simulink model "Just_The_Electrical_model"  (R2016a)
settings: Solver=VariableStepAuto  StartTime=0.0  StopTime=10.0  RelTol=1e-3
values from neighbouring files (symbols this model uses):
  BT = {}    [Electrical_model_settings.m]
  btc = {}    [Electrical_model_settings.m]
  col = {}    [Electrical_model_settings.m]
  elc = {}    [Electrical_model_settings.m]
  ess = {}    [Electrical_model_settings.m]
  fcc = {}    [Electrical_model_settings.m]
  flex = {}    [Electrical_model_settings.m]
  systemBase = {}    [Electrical_model_settings.m]
  wf = {}    [Electrical_model_settings.m]
  wt1 = {}    [Electrical_model_settings.m]
  wt2 = wt1    [Electrical_model_settings.m]
  wt3 = wt1    [Electrical_model_settings.m]
undefined symbols (not defined in the file or in its folder): avr, D1, Delta, DiscIntNeverNeededParam, f2ctrl, governor, interface, Lf1, sm, Ts, Ts_phy, Ts_sim, u0
libraries: powerlib x69, pwrsysBasic x68, simulink_extras x37, pwrsysVICtrl x22, powerlib_meascontrol x19, simulink x8, pwrsysVSrc x5, pwrsysTransf x5, pwrsys-matlab x1
(part 4 of 4)

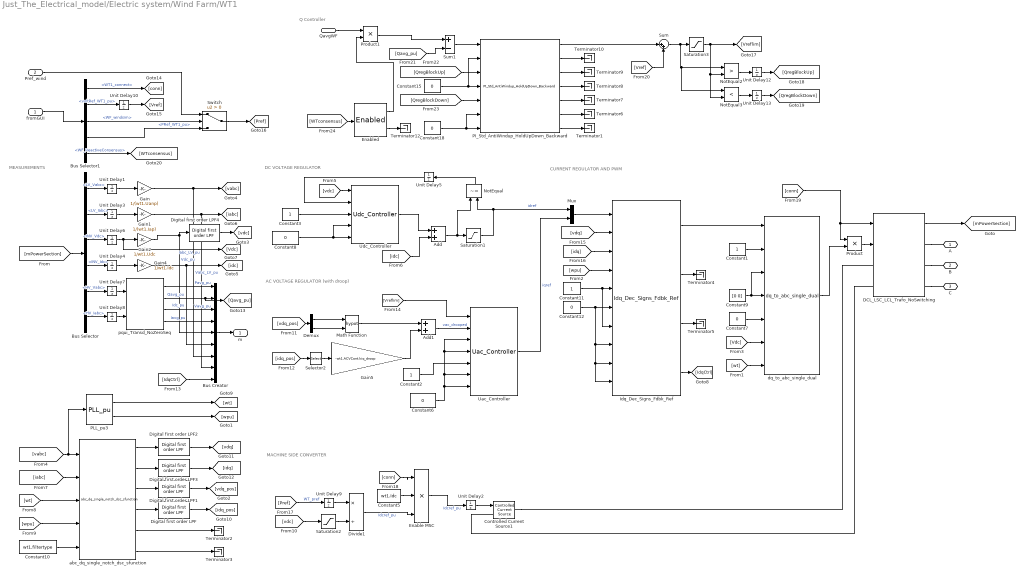
== system Just_The_Electrical_model/Electric system/Wind Farm/WT1 ==
  note: MEASUREMENTS
  note: MACHINE SIDE CONVERTER
  note: AC VOLTAGE REGULATOR (with droop)
  note: DC VOLTAGE REGULATOR
  note: CURRENT REGULATOR AND PWM
  note: Q Controller
  fromGUI : Inport
  Pref_wind : Inport  Port=2
  QavgWF : Inport  Port=3
  Add : Sum
  Add1 : Sum
  Bus Creator : BusCreator  Inputs=9
  Bus Selector : BusSelector  OutputSignals=LV_Vabc,LV_Iabc,INV_Vdc,INV_Idc,HV_Vabc,HV_Iabc
  Bus Selector1 : BusSelector  OutputSignals=WT1_connect,voltRef_WT1_pu,WF_windsim,PRef_WT1_pu,WF_ReactiveConsensus
  Constant1 : Constant  SampleTime=wt1.Ts_control
  Constant10 : Constant  Value=wt1.filtertype  SampleTime=wt1.Ts_control
  Constant11 : Constant  SampleTime=wt2.Ts_control
  Constant12 : Constant  Value=0  SampleTime=wt2.Ts_control
  Constant15 : Constant  Value=0
  Constant18 : Constant  Value=0
  Constant2 : Constant  SampleTime=wt2.Ts_control
  Constant3 : Constant  SampleTime=wt2.Ts_control
  Constant5 : Constant  Value=wt1.Idc  SampleTime=wt1.Ts_control
  Constant6 : Constant  Value=0  SampleTime=wt1.Ts_control
  Constant7 : Constant  Value=0  SampleTime=wt1.Ts_control
  Constant8 : Constant  Value=0  SampleTime=wt1.Ts_control
  Constant9 : Constant  Value=[0 0]  SampleTime=wt1.Ts_control
  Controlled Current Source1 : powerlib/Electrical Sources/Controlled Current Source  Initialize=on  Source_Type=DC  Amplitude=0  Phase=0  Frequency=50  Measurements=None
  DCL_LSC_LCL_Trafo_NoSwitching : pwrsysVSrc/DCL_LSC_LCL_Trafo_NoSwitching  Sn=wt1.Sn  fn=systemBase.fn  Uhv_ab=col.Un  Uab=wt1.Un  lf2=wt1.LCL.l2  rf2=wt1.LCL.r2  Lf1=wt1.LCL.L1  Rf1=wt1.LCL.R1  Cf=wt1.LCL.Cf  Rc=wt1.LCL.Rf  Cdc=wt1.Cdc  Udc0=wt1.Udc  Tsm=wt1.Ts_control  Tstart=wt1.DCVCont.Start
  Demux : Demux  Outputs=2
  Digital first order LPF{,1..4} (5 alike) : pwrsysBasic/Digital first order LPF  Ts=wt1.Ts_control  fcutout=wt1.CurrCont.f_LPF_noise
  Divide1 : Product  Inputs=*/
  Enable MSC : Product  Inputs=3
  Enabled : pwrsysBasic/Enabled
  Gain : Gain  Gain=1/(wt1.Uanp)
  Gain1 : Gain  Gain=1/(wt1.Iap)
  Gain2 : Gain  Gain=1/wt1.Udc
  Gain4 : Gain  Gain=1/wt1.Idc
  Gain5 : Gain  Gain=-wt1.ACVCont.kiq_droop
  Idq_Dec_Signs_Fdbk_Ref : pwrsysVICtrl/Idq_Dec_Signs_Fdbk_Ref  Ts=wt1.Ts_control  fn=systemBase.fn  Kp=wt1.CurrContSingle.kp  Ti=wt1.CurrContSingle.Ti  L=wt1.CurrCont.x  PI_max=wt1.CurrCont.PImax  PI_min=wt1.CurrCont.PImin  TrafoPhaseComp=0
  Math Function : Math  Operator=hypot  SaturateOnIntegerOverflow=on
  Mux : Mux  Inputs=2
  NotEqual : RelationalOperator  Operator=~=  OutDataTypeStr=boolean
  NotEqual2 : RelationalOperator  Operator=>  OutDataTypeStr=boolean
  NotEqual3 : RelationalOperator  Operator=<  OutDataTypeStr=boolean
  PI_Std_AntiWindup_HoldUpDown_Backward : pwrsysBasic/PI_Std_AntiWindup_HoldUpDown_Backward  Ts=wt1.Ts_control  Kg=wt1.Qctrl.Kg  Kp=wt1.Qctrl.Kp  Ti=wt1.Qctrl.Ti  outMax=wt1.Qctrl.deltaUmaxPos  outMin=wt1.Qctrl.deltaUmaxNeg
  PLL_pu3 : pwrsysBasic/PLL_pu  fn=systemBase.fn  Ts=wt1.Ts_control  Kp_pll=90  Ki_pll=1200  Kd_pll=0  PLL_ini=60
  Product : Product
  Product1 : Product
  Saturation1 : Saturate  UpperLimit=wt1.DCVCont.PImax  LowerLimit=wt1.DCVCont.PImin
  Saturation2 : Saturate  UpperLimit=1.2  LowerLimit=0.8
  Saturation3 : Saturate  UpperLimit=wt1.Qctrl.Umax  LowerLimit=wt1.Qctrl.Umin
  Selector2 : Selector  IndexMode=Zero-based  InputPortWidth=2  IndexOptions=Index vector (dialog)  Indices=1  OutputSizes=1
  Sum : Sum  Inputs=|++
  Sum1 : Sum  Inputs=+-
  Switch : Switch  Criteria=u2 > Threshold
  Terminator{1..10,12} (11 alike) : Terminator
  Uac_Controller : pwrsysVICtrl/Uac_Controller  Ts=wt1.Ts_control  Kg=wt1.ACVCont.kg  Kp=wt1.ACVCont.kp  Ti=wt1.ACVCont.Ti  PI_max=wt1.ACVCont.PImax  PI_min=wt1.ACVCont.PImin
  Udc_Controller : pwrsysVICtrl/Udc_Controller  Ts=wt1.Ts_control  Kp=wt1.DCVContSingle.kp  Ti=wt1.DCVContSingle.Ti  PI_max=wt1.DCVCont.PImax  PI_min=wt1.DCVCont.PImin
  Unit Delay{1,3,7..8} (4 alike) : UnitDelay  InitialCondition=[0 0 0]  SampleTime=wt1.Ts_control
  Unit Delay10 : UnitDelay  InitialCondition=1  SampleTime=wt1.Ts_control
  Unit Delay{2,4..5,9,12..13} (6 alike) : UnitDelay  SampleTime=wt1.Ts_control
  Unit Delay6 : UnitDelay  InitialCondition=1  SampleTime=wt1.Ts_control
  abc_dq_single_notch_dsc_sfunction : pwrsysTransf/abc_dq_single_notch_dsc_sfunction  Ts=wt1.Ts_control  fn=2*systemBase.fn  zeta=wt1.CurrCont.zeta
  dq_to_abc_single_dual : pwrsysVICtrl/dq_to_abc_single_dual  Ts=wt1.Ts_control  Uabp=wt1.Uabp
  pqui_Transd_NoZeroSeq : pwrsysBasic/pqui_Transd_NoZeroSeq  Sn=wt1.Sn  Uanp=col.Uanp  Iap=wt1.Iap*(wt1.Un/col.Un)
  A : PMIOPort  Port=1  Side=Right
  B : PMIOPort  Port=2  Side=Right
  C : PMIOPort  Port=3  Side=Right
  m : Outport
  wires:
  Divide1/1 -> Enable MSC/3  "Idcref_pu"
  Bus Selector/1 -> Unit Delay1/1  "<LV_Vabc>"
  [idq_pos] -> Selector2/1
  Unit Delay2/1 -> Controlled Current Source1/1
  Gain1/1 -> Bus Creator/8, [iabc]  "Iabc_LV_pu"
  Bus Selector/2 -> Unit Delay3/1  "<LV_Iabc>"
  Gain5/1 -> Add1/2
  Math Function/1 -> Add1/1
  Constant6/1 -> Uac_Controller/7, Uac_Controller/6, Uac_Controller/3, Uac_Controller/4
  Constant5/1 -> Enable MSC/2
  Add1/1 -> Uac_Controller/2  "vac_drooped"
  [mPowerSection] -> Bus Selector/1
  Enable MSC/1 -> Unit Delay2/1  "Idcref_pu"
  Gain/1 -> Bus Creator/7, [vabc]  "Vabc_LV_pu"
  Constant2/1 -> Uac_Controller/5
  Constant8/1 -> Udc_Controller/4, Udc_Controller/5
  NotEqual/1 -> Unit Delay5/1
  [vdc] -> Udc_Controller/1
  Unit Delay5/1 -> Udc_Controller/2
  Saturation1/1 -> NotEqual/2, Mux/1  "idref"
  [idc] -> Add/2
  Udc_Controller/1 -> Add/1
  Add/1 -> NotEqual/1, Saturation1/1
  Constant3/1 -> Udc_Controller/3
  [idq] -> Idq_Dec_Signs_Fdbk_Ref/3
  [Vdc] -> dq_to_abc_single_dual/6
  [wpu] -> Idq_Dec_Signs_Fdbk_Ref/4
  dq_to_abc_single_dual/1 -> Product/2
  [conn] -> Product/1, DCL_LSC_LCL_Trafo_NoSwitching/1
  Saturation2/1 -> Divide1/2
  [Pref] -> Unit Delay9/1  "WT_pref"
  [vdc] -> Saturation2/1
  [wt] -> dq_to_abc_single_dual/7
  Constant10/1 -> abc_dq_single_notch_dsc_sfunction/5
  Bus Selector/5 -> Unit Delay7/1  "<HV_Vabc>"
  Bus Selector/6 -> Unit Delay8/1  "<HV_Iabc>"
  pqui_Transd_NoZeroSeq/1 -> Bus Creator/1  "Pavg_pu"
  pqui_Transd_NoZeroSeq/2 -> [Qavg_pu], Bus Creator/2  "Qavg_pu"
  pqui_Transd_NoZeroSeq/3 -> Bus Creator/3  "Vavg_pu"
  pqui_Transd_NoZeroSeq/4 -> Bus Creator/4  "Iavg_pu"
  Bus Creator/1 -> m/1
  Bus Selector/3 -> Unit Delay6/1  "<INV_Vdc>"
  Gain2/1 -> Digital first order LPF4/1, Bus Creator/5  "Vdc_pu"
  Gain4/1 -> [idc], Bus Creator/6  "Idc_pu"
  Bus Selector/4 -> Unit Delay4/1  "<INV_Idc>"
  PLL_pu3/2 -> [wpu]
  PLL_pu3/1 -> [wt]
  Uac_Controller/1 -> Mux/2  "iqref"
  DCL_LSC_LCL_Trafo_NoSwitching/1 -> [mPowerSection]
  Unit Delay1/1 -> Gain/1
  Unit Delay3/1 -> Gain1/1
  Unit Delay4/1 -> Gain4/1
  Unit Delay8/1 -> pqui_Transd_NoZeroSeq/2
  Unit Delay6/1 -> [Vdc], Gain2/1
  Unit Delay7/1 -> pqui_Transd_NoZeroSeq/1
  Unit Delay9/1 -> Divide1/1
  [Vreflim] -> Uac_Controller/1
  abc_dq_single_notch_dsc_sfunction/6 -> Terminator3/1
  abc_dq_single_notch_dsc_sfunction/5 -> Terminator2/1
  Selector2/1 -> Gain5/1
  Idq_Dec_Signs_Fdbk_Ref/2 -> Terminator4/1
  [vdq] -> Idq_Dec_Signs_Fdbk_Ref/2
  Constant1/1 -> dq_to_abc_single_dual/2
  Constant7/1 -> dq_to_abc_single_dual/5
  Constant9/1 -> dq_to_abc_single_dual/4, dq_to_abc_single_dual/3
  Constant11/1 -> Idq_Dec_Signs_Fdbk_Ref/7, Idq_Dec_Signs_Fdbk_Ref/5
  Constant12/1 -> Idq_Dec_Signs_Fdbk_Ref/8, Idq_Dec_Signs_Fdbk_Ref/9, Idq_Dec_Signs_Fdbk_Ref/10, Idq_Dec_Signs_Fdbk_Ref/6
  Idq_Dec_Signs_Fdbk_Ref/3 -> Terminator5/1
  Idq_Dec_Signs_Fdbk_Ref/4 -> [IdqCtrl]
  [IdqCtrl] -> Bus Creator/9
  Idq_Dec_Signs_Fdbk_Ref/1 -> dq_to_abc_single_dual/1
  [wt] -> abc_dq_single_notch_dsc_sfunction/3
  [wpu] -> abc_dq_single_notch_dsc_sfunction/4
  abc_dq_single_notch_dsc_sfunction/1 -> Digital first order LPF2/1
  [vabc] -> abc_dq_single_notch_dsc_sfunction/1, PLL_pu3/1
  [iabc] -> abc_dq_single_notch_dsc_sfunction/2
  abc_dq_single_notch_dsc_sfunction/3 -> Digital first order LPF1/1
  abc_dq_single_notch_dsc_sfunction/4 -> Digital first order LPF/1
  abc_dq_single_notch_dsc_sfunction/2 -> Digital first order LPF3/1
  Digital first order LPF/1 -> [idq_pos]
  Digital first order LPF1/1 -> [vdq_pos]
  [vdq_pos] -> Demux/1
  Demux/1 -> Math Function/1
  Demux/2 -> Math Function/2
  Digital first order LPF2/1 -> [vdq]
  Digital first order LPF3/1 -> [idq]
  Digital first order LPF4/1 -> [vdc]
  fromGUI/1 -> Bus Selector1/1
  Bus Selector1/4 -> Switch/3  "<PRef_WT1_pu>"
  Bus Selector1/1 -> [conn]  "<WT1_connect>"
  Bus Selector1/2 -> Unit Delay10/1  "<voltRef_WT1_pu>"
  [conn] -> Enable MSC/1
  Pref_wind/1 -> Switch/1
  Bus Selector1/3 -> Switch/2  "<WF_windsim>"
  Switch/1 -> [Pref]
  Mux/1 -> Idq_Dec_Signs_Fdbk_Ref/1
  Product/1 -> DCL_LSC_LCL_Trafo_NoSwitching/2
  Unit Delay10/1 -> [Vref]
  [Vref] -> Sum/2
  Sum/1 -> NotEqual3/1, NotEqual2/1, Saturation3/1
  Saturation3/1 -> NotEqual3/2, NotEqual2/2, [Vreflim]
  [Qavg_pu] -> Sum1/2
  [WTconsensus] -> Enabled/1
  [QregBlockUp] -> PI_Std_AntiWindup_HoldUpDown_Backward/3
  Constant15/1 -> PI_Std_AntiWindup_HoldUpDown_Backward/2, PI_Std_AntiWindup_HoldUpDown_Backward/4
  [QregBlockDown] -> PI_Std_AntiWindup_HoldUpDown_Backward/5
  Constant18/1 -> PI_Std_AntiWindup_HoldUpDown_Backward/6, PI_Std_AntiWindup_HoldUpDown_Backward/7
  PI_Std_AntiWindup_HoldUpDown_Backward/7 -> Terminator1/1
  PI_Std_AntiWindup_HoldUpDown_Backward/6 -> Terminator6/1
  PI_Std_AntiWindup_HoldUpDown_Backward/5 -> Terminator7/1
  PI_Std_AntiWindup_HoldUpDown_Backward/4 -> Terminator8/1
  PI_Std_AntiWindup_HoldUpDown_Backward/3 -> Terminator9/1
  PI_Std_AntiWindup_HoldUpDown_Backward/2 -> Terminator10/1
  NotEqual2/1 -> Unit Delay12/1
  Unit Delay12/1 -> [QregBlockUp]
  NotEqual3/1 -> Unit Delay13/1
  Unit Delay13/1 -> [QregBlockDown]
  PI_Std_AntiWindup_HoldUpDown_Backward/1 -> Sum/1
  Bus Selector1/5 -> [WTconsensus]  "<WF_ReactiveConsensus>"
  Sum1/1 -> PI_Std_AntiWindup_HoldUpDown_Backward/1
  Enabled/2 -> Terminator12/1
  QavgWF/1 -> Product1/1
  Product1/1 -> Sum1/1
  Enabled/1 -> Product1/2
  connections:
  Controlled Current Source1/RConn1 -- DCL_LSC_LCL_Trafo_NoSwitching/LConn1
  DCL_LSC_LCL_Trafo_NoSwitching/RConn3 -- C/RConn1
  DCL_LSC_LCL_Trafo_NoSwitching/RConn1 -- A/RConn1
  DCL_LSC_LCL_Trafo_NoSwitching/RConn2 -- B/RConn1
  Controlled Current Source1/LConn1 -- DCL_LSC_LCL_Trafo_NoSwitching/LConn2

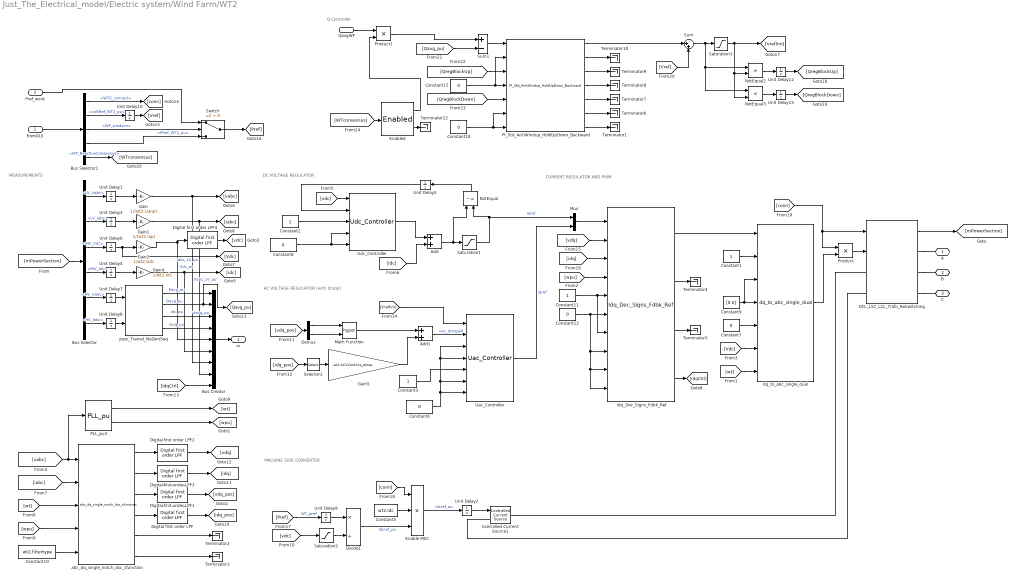
== system Just_The_Electrical_model/Electric system/Wind Farm/WT2 ==
  note: MEASUREMENTS
  note: MACHINE SIDE CONVERTER
  note: AC VOLTAGE REGULATOR (with droop)
  note: DC VOLTAGE REGULATOR
  note: CURRENT REGULATOR AND PWM
  note: Q Controller
  fromGUI : Inport
  Pref_wind : Inport  Port=2
  QavgWF : Inport  Port=3
  Add : Sum
  Add1 : Sum
  Bus Creator : BusCreator  Inputs=9
  Bus Selector : BusSelector  OutputSignals=LV_Vabc,LV_Iabc,INV_Vdc,INV_Idc,HV_Vabc,HV_Iabc
  Bus Selector1 : BusSelector  OutputSignals=WT2_connect,voltRef_WT2_pu,WF_windsim,PRef_WT2_pu,WF_ReactiveConsensus
  Constant{1..3,11} (4 alike) : Constant  SampleTime=wt2.Ts_control
  Constant10 : Constant  Value=wt2.filtertype  SampleTime=wt2.Ts_control
  Constant{6..8,12} (4 alike) : Constant  Value=0  SampleTime=wt2.Ts_control
  Constant15 : Constant  Value=0
  Constant18 : Constant  Value=0
  Constant5 : Constant  Value=wt2.Idc  SampleTime=wt2.Ts_control
  Constant9 : Constant  Value=[0 0]  SampleTime=wt2.Ts_control
  Controlled Current Source1 : powerlib/Electrical Sources/Controlled Current Source  Initialize=on  Source_Type=DC  Amplitude=0  Phase=0  Frequency=50  Measurements=None
  DCL_LSC_LCL_Trafo_NoSwitching : pwrsysVSrc/DCL_LSC_LCL_Trafo_NoSwitching  Sn=wt2.Sn  fn=systemBase.fn  Uhv_ab=col.Un  Uab=wt2.Un  lf2=wt2.LCL.l2  rf2=wt2.LCL.r2  Lf1=wt2.LCL.L1  Rf1=wt2.LCL.R1  Cf=wt2.LCL.Cf  Rc=wt2.LCL.Rf  Cdc=wt2.Cdc  Udc0=wt2.Udc  Tsm=wt2.Ts_control  Tstart=wt2.DCVCont.Start
  Demux : Demux  Outputs=2
  Digital first order LPF{,1..4} (5 alike) : pwrsysBasic/Digital first order LPF  Ts=wt2.Ts_control  fcutout=wt2.CurrCont.f_LPF_noise
  Divide1 : Product  Inputs=*/
  Enable MSC : Product  Inputs=3
  Enabled : pwrsysBasic/Enabled
  Gain : Gain  Gain=1/(wt2.Uanp)
  Gain1 : Gain  Gain=1/(wt2.Iap)
  Gain2 : Gain  Gain=1/wt2.Udc
  Gain4 : Gain  Gain=1/wt2.Idc
  Gain5 : Gain  Gain=-wt2.ACVCont.kiq_droop
  Idq_Dec_Signs_Fdbk_Ref : pwrsysVICtrl/Idq_Dec_Signs_Fdbk_Ref  Ts=wt2.Ts_control  fn=systemBase.fn  Kp=wt2.CurrContSingle.kp  Ti=wt2.CurrContSingle.Ti  L=wt2.CurrCont.x  PI_max=wt2.CurrCont.PImax  PI_min=wt2.CurrCont.PImin  TrafoPhaseComp=0
  Math Function : Math  Operator=hypot  SaturateOnIntegerOverflow=on
  Mux : Mux  Inputs=2
  NotEqual : RelationalOperator  Operator=~=  OutDataTypeStr=boolean
  NotEqual2 : RelationalOperator  Operator=>  OutDataTypeStr=boolean
  NotEqual3 : RelationalOperator  Operator=<  OutDataTypeStr=boolean
  PI_Std_AntiWindup_HoldUpDown_Backward : pwrsysBasic/PI_Std_AntiWindup_HoldUpDown_Backward  Ts=wt2.Ts_control  Kg=wt2.Qctrl.Kg  Kp=wt2.Qctrl.Kp  Ti=wt2.Qctrl.Ti  outMax=wt2.Qctrl.deltaUmaxPos  outMin=wt2.Qctrl.deltaUmaxNeg
  PLL_pu3 : pwrsysBasic/PLL_pu  fn=systemBase.fn  Ts=wt2.Ts_control  Kp_pll=90  Ki_pll=1200  Kd_pll=0  PLL_ini=60
  Product : Product
  Product1 : Product
  Saturation1 : Saturate  UpperLimit=wt2.DCVCont.PImax  LowerLimit=wt2.DCVCont.PImin
  Saturation2 : Saturate  UpperLimit=1.2  LowerLimit=0.8
  Saturation3 : Saturate  UpperLimit=wt2.Qctrl.Umax  LowerLimit=wt2.Qctrl.Umin
  Selector2 : Selector  IndexMode=Zero-based  InputPortWidth=2  IndexOptions=Index vector (dialog)  Indices=1  OutputSizes=1
  Sum : Sum  Inputs=|++
  Sum1 : Sum  Inputs=+-
  Switch : Switch  Criteria=u2 > Threshold
  Terminator{1..10,12} (11 alike) : Terminator
  Uac_Controller : pwrsysVICtrl/Uac_Controller  Ts=wt2.Ts_control  Kg=wt2.ACVCont.kg  Kp=wt2.ACVCont.kp  Ti=wt2.ACVCont.Ti  PI_max=wt2.ACVCont.PImax  PI_min=wt2.ACVCont.PImin
  Udc_Controller : pwrsysVICtrl/Udc_Controller  Ts=wt2.Ts_control  Kp=wt2.DCVContDual.kp  Ti=wt2.DCVContDual.Ti  PI_max=wt2.DCVCont.PImax  PI_min=wt2.DCVCont.PImin
  Unit Delay{1,3,7..8} (4 alike) : UnitDelay  InitialCondition=[0 0 0]  SampleTime=wt2.Ts_control
  Unit Delay10 : UnitDelay  InitialCondition=1  SampleTime=wt2.Ts_control
  Unit Delay{2,4..5,9,12..13} (6 alike) : UnitDelay  SampleTime=wt2.Ts_control
  Unit Delay6 : UnitDelay  InitialCondition=1  SampleTime=wt2.Ts_control
  abc_dq_single_notch_dsc_sfunction : pwrsysTransf/abc_dq_single_notch_dsc_sfunction  Ts=wt2.Ts_control  fn=2*systemBase.fn  zeta=wt2.CurrCont.zeta
  dq_to_abc_single_dual : pwrsysVICtrl/dq_to_abc_single_dual  Ts=wt2.Ts_control  Uabp=wt2.Uabp
  pqui_Transd_NoZeroSeq : pwrsysBasic/pqui_Transd_NoZeroSeq  Sn=wt2.Sn  Uanp=col.Uanp  Iap=wt2.Iap*(wt2.Un/col.Un)
  A : PMIOPort  Port=1  Side=Right
  B : PMIOPort  Port=2  Side=Right
  C : PMIOPort  Port=3  Side=Right
  m : Outport
  wires:
  Divide1/1 -> Enable MSC/3  "Idcref_pu"
  Bus Selector/1 -> Unit Delay1/1  "<LV_Vabc>"
  [idq_pos] -> Selector2/1
  Unit Delay2/1 -> Controlled Current Source1/1
  Gain1/1 -> Bus Creator/8, [iabc]  "Iabc_LV_pu"
  Bus Selector/2 -> Unit Delay3/1  "<LV_Iabc>"
  Gain5/1 -> Add1/2
  Math Function/1 -> Add1/1
  Constant6/1 -> Uac_Controller/7, Uac_Controller/6, Uac_Controller/3, Uac_Controller/4
  Constant5/1 -> Enable MSC/2
  Add1/1 -> Uac_Controller/2  "vac_drooped"
  [mPowerSection] -> Bus Selector/1
  Enable MSC/1 -> Unit Delay2/1  "Idcref_pu"
  Gain/1 -> Bus Creator/7, [vabc]  "Vabc_LV_pu"
  Constant3/1 -> Uac_Controller/5
  Constant8/1 -> Udc_Controller/4, Udc_Controller/5
  NotEqual/1 -> Unit Delay5/1
  [vdc] -> Udc_Controller/1
  Unit Delay5/1 -> Udc_Controller/2
  Saturation1/1 -> NotEqual/2, Mux/1  "idref"
  [idc] -> Add/2
  Udc_Controller/1 -> Add/1
  Add/1 -> NotEqual/1, Saturation1/1
  Constant2/1 -> Udc_Controller/3
  [idq] -> Idq_Dec_Signs_Fdbk_Ref/3
  [Vdc] -> dq_to_abc_single_dual/6
  [wpu] -> Idq_Dec_Signs_Fdbk_Ref/4
  dq_to_abc_single_dual/1 -> Product/2
  Mux/1 -> Idq_Dec_Signs_Fdbk_Ref/1
  [conn] -> Product/1, DCL_LSC_LCL_Trafo_NoSwitching/1
  Saturation2/1 -> Divide1/2
  [Pref] -> Unit Delay9/1  "WT_pref"
  [vdc] -> Saturation2/1
  [wt] -> dq_to_abc_single_dual/7
  Constant10/1 -> abc_dq_single_notch_dsc_sfunction/5
  Bus Selector/5 -> Unit Delay7/1  "<HV_Vabc>"
  Bus Selector/6 -> Unit Delay8/1  "<HV_Iabc>"
  pqui_Transd_NoZeroSeq/1 -> Bus Creator/1  "Pavg_pu"
  pqui_Transd_NoZeroSeq/2 -> [Qavg_pu], Bus Creator/2  "Qavg_pu"
  pqui_Transd_NoZeroSeq/3 -> Bus Creator/3  "Vavg_pu"
  pqui_Transd_NoZeroSeq/4 -> Bus Creator/4  "Iavg_pu"
  Bus Creator/1 -> m/1
  Bus Selector/3 -> Unit Delay6/1  "<INV_Vdc>"
  Gain2/1 -> Bus Creator/5, Digital first order LPF4/1  "Vdc_pu"
  Gain4/1 -> [idc], Bus Creator/6  "Idc_pu"
  Bus Selector/4 -> Unit Delay4/1  "<INV_Idc>"
  PLL_pu3/2 -> [wpu]
  PLL_pu3/1 -> [wt]
  Uac_Controller/1 -> Mux/2  "iqref"
  DCL_LSC_LCL_Trafo_NoSwitching/1 -> [mPowerSection]
  Unit Delay1/1 -> Gain/1
  Unit Delay3/1 -> Gain1/1
  Unit Delay4/1 -> Gain4/1
  Unit Delay8/1 -> pqui_Transd_NoZeroSeq/2
  Unit Delay6/1 -> [Vdc], Gain2/1
  Unit Delay7/1 -> pqui_Transd_NoZeroSeq/1
  Unit Delay9/1 -> Divide1/1
  [Vreflim] -> Uac_Controller/1
  abc_dq_single_notch_dsc_sfunction/6 -> Terminator3/1
  abc_dq_single_notch_dsc_sfunction/5 -> Terminator2/1
  Selector2/1 -> Gain5/1
  Idq_Dec_Signs_Fdbk_Ref/2 -> Terminator4/1
  [vdq] -> Idq_Dec_Signs_Fdbk_Ref/2
  Constant1/1 -> dq_to_abc_single_dual/2
  Constant7/1 -> dq_to_abc_single_dual/5
  Constant9/1 -> dq_to_abc_single_dual/4, dq_to_abc_single_dual/3
  Constant11/1 -> Idq_Dec_Signs_Fdbk_Ref/7, Idq_Dec_Signs_Fdbk_Ref/5
  Constant12/1 -> Idq_Dec_Signs_Fdbk_Ref/8, Idq_Dec_Signs_Fdbk_Ref/9, Idq_Dec_Signs_Fdbk_Ref/10, Idq_Dec_Signs_Fdbk_Ref/6
  Idq_Dec_Signs_Fdbk_Ref/3 -> Terminator5/1
  Idq_Dec_Signs_Fdbk_Ref/4 -> [IdqCtrl]
  [IdqCtrl] -> Bus Creator/9
  Idq_Dec_Signs_Fdbk_Ref/1 -> dq_to_abc_single_dual/1
  [wt] -> abc_dq_single_notch_dsc_sfunction/3
  [wpu] -> abc_dq_single_notch_dsc_sfunction/4
  abc_dq_single_notch_dsc_sfunction/1 -> Digital first order LPF2/1
  [vabc] -> abc_dq_single_notch_dsc_sfunction/1, PLL_pu3/1
  [iabc] -> abc_dq_single_notch_dsc_sfunction/2
  abc_dq_single_notch_dsc_sfunction/3 -> Digital first order LPF1/1
  abc_dq_single_notch_dsc_sfunction/4 -> Digital first order LPF/1
  abc_dq_single_notch_dsc_sfunction/2 -> Digital first order LPF3/1
  Digital first order LPF/1 -> [idq_pos]
  Digital first order LPF1/1 -> [vdq_pos]
  [vdq_pos] -> Demux/1
  Demux/1 -> Math Function/1
  Demux/2 -> Math Function/2
  Digital first order LPF2/1 -> [vdq]
  Digital first order LPF3/1 -> [idq]
  Digital first order LPF4/1 -> [vdc]
  fromGUI/1 -> Bus Selector1/1
  Bus Selector1/4 -> Switch/3  "<PRef_WT2_pu>"
  Bus Selector1/1 -> [conn]  "<WT2_connect>"
  Bus Selector1/2 -> Unit Delay10/1  "<voltRef_WT2_pu>"
  [conn] -> Enable MSC/1
  Pref_wind/1 -> Switch/1
  Bus Selector1/3 -> Switch/2  "<WF_windsim>"
  Switch/1 -> [Pref]
  Product/1 -> DCL_LSC_LCL_Trafo_NoSwitching/2
  Unit Delay10/1 -> [Vref]
  [Vref] -> Sum/2
  Sum/1 -> NotEqual3/1, NotEqual2/1, Saturation3/1
  Saturation3/1 -> NotEqual3/2, NotEqual2/2, [Vreflim]
  [Qavg_pu] -> Sum1/2
  [WTconsensus] -> Enabled/1
  [QregBlockUp] -> PI_Std_AntiWindup_HoldUpDown_Backward/3
  Constant15/1 -> PI_Std_AntiWindup_HoldUpDown_Backward/2, PI_Std_AntiWindup_HoldUpDown_Backward/4
  [QregBlockDown] -> PI_Std_AntiWindup_HoldUpDown_Backward/5
  Constant18/1 -> PI_Std_AntiWindup_HoldUpDown_Backward/6, PI_Std_AntiWindup_HoldUpDown_Backward/7
  PI_Std_AntiWindup_HoldUpDown_Backward/7 -> Terminator1/1
  PI_Std_AntiWindup_HoldUpDown_Backward/6 -> Terminator6/1
  PI_Std_AntiWindup_HoldUpDown_Backward/5 -> Terminator7/1
  PI_Std_AntiWindup_HoldUpDown_Backward/4 -> Terminator8/1
  PI_Std_AntiWindup_HoldUpDown_Backward/3 -> Terminator9/1
  PI_Std_AntiWindup_HoldUpDown_Backward/2 -> Terminator10/1
  NotEqual2/1 -> Unit Delay12/1
  Unit Delay12/1 -> [QregBlockUp]
  NotEqual3/1 -> Unit Delay13/1
  Unit Delay13/1 -> [QregBlockDown]
  PI_Std_AntiWindup_HoldUpDown_Backward/1 -> Sum/1
  Bus Selector1/5 -> [WTconsensus]  "<WF_ReactiveConsensus>"
  Sum1/1 -> PI_Std_AntiWindup_HoldUpDown_Backward/1
  Enabled/2 -> Terminator12/1
  QavgWF/1 -> Product1/1
  Product1/1 -> Sum1/1
  Enabled/1 -> Product1/2
  connections:
  Controlled Current Source1/RConn1 -- DCL_LSC_LCL_Trafo_NoSwitching/LConn1
  DCL_LSC_LCL_Trafo_NoSwitching/RConn3 -- C/RConn1
  DCL_LSC_LCL_Trafo_NoSwitching/RConn1 -- A/RConn1
  DCL_LSC_LCL_Trafo_NoSwitching/RConn2 -- B/RConn1
  Controlled Current Source1/LConn1 -- DCL_LSC_LCL_Trafo_NoSwitching/LConn2

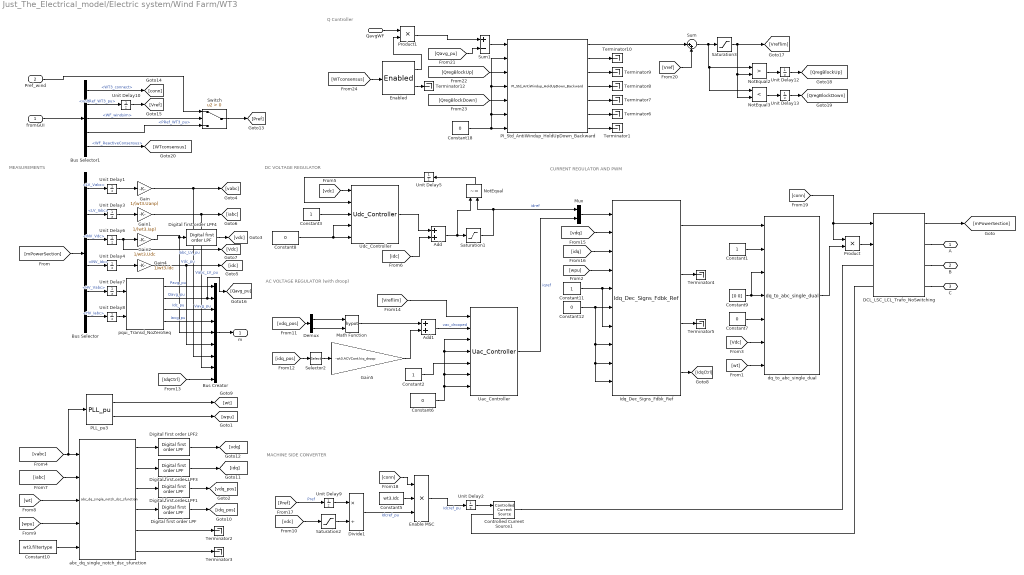
== system Just_The_Electrical_model/Electric system/Wind Farm/WT3 ==
  note: Q Controller
  note: MEASUREMENTS
  note: MACHINE SIDE CONVERTER
  note: AC VOLTAGE REGULATOR (with droop)
  note: DC VOLTAGE REGULATOR
  note: CURRENT REGULATOR AND PWM
  fromGUI : Inport
  Pref_wind : Inport  Port=2
  QavgWF : Inport  Port=3
  Add : Sum
  Add1 : Sum
  Bus Creator : BusCreator  Inputs=9
  Bus Selector : BusSelector  OutputSignals=LV_Vabc,LV_Iabc,INV_Vdc,INV_Idc,HV_Vabc,HV_Iabc
  Bus Selector1 : BusSelector  OutputSignals=WT3_connect,voltRef_WT3_pu,WF_windsim,PRef_WT3_pu,WF_ReactiveConsensus
  Constant1 : Constant  SampleTime=wt3.Ts_control
  Constant10 : Constant  Value=wt3.filtertype  SampleTime=wt3.Ts_control
  Constant11 : Constant  SampleTime=wt3.Ts_control
  Constant{6..8,12} (4 alike) : Constant  Value=0  SampleTime=wt3.Ts_control
  Constant18 : Constant  Value=0
  Constant2 : Constant  SampleTime=wt2.Ts_control
  Constant3 : Constant  SampleTime=wt2.Ts_control
  Constant5 : Constant  Value=wt3.Idc  SampleTime=wt3.Ts_control
  Constant9 : Constant  Value=[0 0]  SampleTime=wt3.Ts_control
  Controlled Current Source1 : powerlib/Electrical Sources/Controlled Current Source  Initialize=on  Source_Type=DC  Amplitude=0  Phase=0  Frequency=50  Measurements=None
  DCL_LSC_LCL_Trafo_NoSwitching : pwrsysVSrc/DCL_LSC_LCL_Trafo_NoSwitching  Sn=wt3.Sn  fn=systemBase.fn  Uhv_ab=col.Un  Uab=wt3.Un  lf2=wt3.LCL.l2  rf2=wt3.LCL.r2  Lf1=wt3.LCL.L1  Rf1=wt3.LCL.R1  Cf=wt3.LCL.Cf  Rc=wt3.LCL.Rf  Cdc=wt3.Cdc  Udc0=wt3.Udc  Tsm=wt3.Ts_control  Tstart=wt3.DCVCont.Start
  Demux : Demux  Outputs=2
  Digital first order LPF{,1..4} (5 alike) : pwrsysBasic/Digital first order LPF  Ts=wt3.Ts_control  fcutout=wt3.CurrCont.f_LPF_noise
  Divide1 : Product  Inputs=*/
  Enable MSC : Product  Inputs=***
  Enabled : pwrsysBasic/Enabled
  Gain : Gain  Gain=1/(wt3.Uanp)
  Gain1 : Gain  Gain=1/(wt3.Iap)
  Gain2 : Gain  Gain=1/wt3.Udc
  Gain4 : Gain  Gain=1/wt3.Idc
  Gain5 : Gain  Gain=-wt3.ACVCont.kiq_droop
  Idq_Dec_Signs_Fdbk_Ref : pwrsysVICtrl/Idq_Dec_Signs_Fdbk_Ref  Ts=wt3.Ts_control  fn=systemBase.fn  Kp=wt3.CurrContSingle.kp  Ti=wt3.CurrContSingle.Ti  L=wt3.CurrCont.x  PI_max=wt3.CurrCont.PImax  PI_min=wt3.CurrCont.PImin  TrafoPhaseComp=0
  Math Function : Math  Operator=hypot  SaturateOnIntegerOverflow=on
  Mux : Mux  Inputs=2
  NotEqual : RelationalOperator  Operator=~=  OutDataTypeStr=boolean
  NotEqual2 : RelationalOperator  Operator=>  OutDataTypeStr=boolean
  NotEqual3 : RelationalOperator  Operator=<  OutDataTypeStr=boolean
  PI_Std_AntiWindup_HoldUpDown_Backward : pwrsysBasic/PI_Std_AntiWindup_HoldUpDown_Backward  Ts=wt3.Ts_control  Kg=wt3.Qctrl.Kg  Kp=wt3.Qctrl.Kp  Ti=wt3.Qctrl.Ti  outMax=wt3.Qctrl.deltaUmaxPos  outMin=wt3.Qctrl.deltaUmaxNeg
  PLL_pu3 : pwrsysBasic/PLL_pu  fn=systemBase.fn  Ts=wt3.Ts_control  Kp_pll=90  Ki_pll=1200  Kd_pll=0  PLL_ini=60
  Product : Product
  Product1 : Product
  Saturation1 : Saturate  UpperLimit=wt3.DCVCont.PImax  LowerLimit=wt3.DCVCont.PImin
  Saturation2 : Saturate  UpperLimit=1.2  LowerLimit=0.8
  Saturation3 : Saturate  UpperLimit=wt3.Qctrl.Umax  LowerLimit=wt3.Qctrl.Umin
  Selector2 : Selector  IndexMode=Zero-based  InputPortWidth=2  IndexOptions=Index vector (dialog)  Indices=1  OutputSizes=1
  Sum : Sum  Inputs=|++
  Sum1 : Sum  Inputs=+-
  Switch : Switch  Criteria=u2 > Threshold
  Terminator{1..10,12} (11 alike) : Terminator
  Uac_Controller : pwrsysVICtrl/Uac_Controller  Ts=wt3.Ts_control  Kg=wt3.ACVCont.kg  Kp=wt3.ACVCont.kp  Ti=wt3.ACVCont.Ti  PI_max=wt3.ACVCont.PImax  PI_min=wt3.ACVCont.PImin
  Udc_Controller : pwrsysVICtrl/Udc_Controller  Ts=wt3.Ts_control  Kp=wt3.DCVContDual.kp  Ti=wt3.DCVContDual.Ti  PI_max=wt3.DCVCont.PImax  PI_min=wt3.DCVCont.PImin
  Unit Delay{1,3,7..8} (4 alike) : UnitDelay  InitialCondition=[0 0 0]  SampleTime=wt3.Ts_control
  Unit Delay10 : UnitDelay  InitialCondition=1  SampleTime=wt3.Ts_control
  Unit Delay{2,4..5,9,12..13} (6 alike) : UnitDelay  SampleTime=wt3.Ts_control
  Unit Delay6 : UnitDelay  InitialCondition=1  SampleTime=wt3.Ts_control
  abc_dq_single_notch_dsc_sfunction : pwrsysTransf/abc_dq_single_notch_dsc_sfunction  Ts=wt3.Ts_control  fn=2*systemBase.fn  zeta=wt3.CurrCont.zeta
  dq_to_abc_single_dual : pwrsysVICtrl/dq_to_abc_single_dual  Ts=wt3.Ts_control  Uabp=wt3.Uabp
  pqui_Transd_NoZeroSeq : pwrsysBasic/pqui_Transd_NoZeroSeq  Sn=wt3.Sn  Uanp=col.Uanp  Iap=wt3.Iap*(wt3.Un/col.Un)
  A : PMIOPort  Port=1  Side=Right
  B : PMIOPort  Port=2  Side=Right
  C : PMIOPort  Port=3  Side=Right
  m : Outport
  wires:
  Divide1/1 -> Enable MSC/3  "Idcref_pu"
  Bus Selector/1 -> Unit Delay1/1  "<LV_Vabc>"
  [idq_pos] -> Selector2/1
  Unit Delay2/1 -> Controlled Current Source1/1
  Gain1/1 -> Bus Creator/8, [iabc]  "Iabc_LV_pu"
  Bus Selector/2 -> Unit Delay3/1  "<LV_Iabc>"
  Gain5/1 -> Add1/2
  Math Function/1 -> Add1/1
  Constant6/1 -> Uac_Controller/7, Uac_Controller/6, Uac_Controller/3, Uac_Controller/4
  Constant5/1 -> Enable MSC/2
  Add1/1 -> Uac_Controller/2  "vac_drooped"
  [mPowerSection] -> Bus Selector/1
  Enable MSC/1 -> Unit Delay2/1  "Idcref_pu"
  Gain/1 -> Bus Creator/7, [vabc]  "Vabc_LV_pu"
  Constant2/1 -> Uac_Controller/5
  Constant8/1 -> Udc_Controller/4, Udc_Controller/5
  NotEqual/1 -> Unit Delay5/1
  [vdc] -> Udc_Controller/1
  Unit Delay5/1 -> Udc_Controller/2
  Saturation1/1 -> NotEqual/2, Mux/1  "idref"
  [idc] -> Add/2
  Udc_Controller/1 -> Add/1
  Add/1 -> NotEqual/1, Saturation1/1
  Constant3/1 -> Udc_Controller/3
  [idq] -> Idq_Dec_Signs_Fdbk_Ref/3
  [Vdc] -> dq_to_abc_single_dual/6
  [wpu] -> Idq_Dec_Signs_Fdbk_Ref/4
  dq_to_abc_single_dual/1 -> Product/2
  Mux/1 -> Idq_Dec_Signs_Fdbk_Ref/1
  [conn] -> Product/1, DCL_LSC_LCL_Trafo_NoSwitching/1
  Saturation2/1 -> Divide1/2
  [Pref] -> Unit Delay9/1  "Pref"
  [vdc] -> Saturation2/1
  [wt] -> dq_to_abc_single_dual/7
  Constant10/1 -> abc_dq_single_notch_dsc_sfunction/5
  Bus Selector/5 -> Unit Delay7/1  "<HV_Vabc>"
  Bus Selector/6 -> Unit Delay8/1  "<HV_Iabc>"
  pqui_Transd_NoZeroSeq/1 -> Bus Creator/1  "Pavg_pu"
  pqui_Transd_NoZeroSeq/2 -> [Qavg_pu], Bus Creator/2  "Qavg_pu"
  pqui_Transd_NoZeroSeq/3 -> Bus Creator/3  "Vavg_pu"
  pqui_Transd_NoZeroSeq/4 -> Bus Creator/4  "Iavg_pu"
  Bus Creator/1 -> m/1
  Bus Selector/3 -> Unit Delay6/1  "<INV_Vdc>"
  Gain2/1 -> Digital first order LPF4/1, Bus Creator/5  "Vdc_pu"
  Gain4/1 -> [idc], Bus Creator/6  "Idc_pu"
  Bus Selector/4 -> Unit Delay4/1  "<INV_Idc>"
  PLL_pu3/2 -> [wpu]
  PLL_pu3/1 -> [wt]
  Uac_Controller/1 -> Mux/2  "iqref"
  DCL_LSC_LCL_Trafo_NoSwitching/1 -> [mPowerSection]
  Unit Delay1/1 -> Gain/1
  Unit Delay3/1 -> Gain1/1
  Unit Delay4/1 -> Gain4/1
  Unit Delay8/1 -> pqui_Transd_NoZeroSeq/2
  Unit Delay6/1 -> [Vdc], Gain2/1
  Unit Delay7/1 -> pqui_Transd_NoZeroSeq/1
  Unit Delay9/1 -> Divide1/1
  [Vreflim] -> Uac_Controller/1
  abc_dq_single_notch_dsc_sfunction/6 -> Terminator3/1
  abc_dq_single_notch_dsc_sfunction/5 -> Terminator2/1
  Selector2/1 -> Gain5/1
  Idq_Dec_Signs_Fdbk_Ref/2 -> Terminator4/1
  [vdq] -> Idq_Dec_Signs_Fdbk_Ref/2
  Constant1/1 -> dq_to_abc_single_dual/2
  Constant7/1 -> dq_to_abc_single_dual/5
  Constant9/1 -> dq_to_abc_single_dual/4, dq_to_abc_single_dual/3
  Constant11/1 -> Idq_Dec_Signs_Fdbk_Ref/7, Idq_Dec_Signs_Fdbk_Ref/5
  Constant12/1 -> Idq_Dec_Signs_Fdbk_Ref/8, Idq_Dec_Signs_Fdbk_Ref/9, Idq_Dec_Signs_Fdbk_Ref/10, Idq_Dec_Signs_Fdbk_Ref/6
  Idq_Dec_Signs_Fdbk_Ref/3 -> Terminator5/1
  Idq_Dec_Signs_Fdbk_Ref/4 -> [IdqCtrl]
  [IdqCtrl] -> Bus Creator/9
  Idq_Dec_Signs_Fdbk_Ref/1 -> dq_to_abc_single_dual/1
  [wt] -> abc_dq_single_notch_dsc_sfunction/3
  [wpu] -> abc_dq_single_notch_dsc_sfunction/4
  abc_dq_single_notch_dsc_sfunction/1 -> Digital first order LPF2/1
  [vabc] -> abc_dq_single_notch_dsc_sfunction/1, PLL_pu3/1
  [iabc] -> abc_dq_single_notch_dsc_sfunction/2
  abc_dq_single_notch_dsc_sfunction/3 -> Digital first order LPF1/1
  abc_dq_single_notch_dsc_sfunction/4 -> Digital first order LPF/1
  abc_dq_single_notch_dsc_sfunction/2 -> Digital first order LPF3/1
  Digital first order LPF/1 -> [idq_pos]
  Digital first order LPF1/1 -> [vdq_pos]
  [vdq_pos] -> Demux/1
  Demux/1 -> Math Function/1
  Demux/2 -> Math Function/2
  Digital first order LPF2/1 -> [vdq]
  Digital first order LPF3/1 -> [idq]
  Digital first order LPF4/1 -> [vdc]
  fromGUI/1 -> Bus Selector1/1
  Bus Selector1/4 -> Switch/3  "<PRef_WT3_pu>"
  Bus Selector1/1 -> [conn]  "<WT3_connect>"
  Bus Selector1/2 -> Unit Delay10/1  "<voltRef_WT3_pu>"
  [conn] -> Enable MSC/1
  Pref_wind/1 -> Switch/1
  Bus Selector1/3 -> Switch/2  "<WF_windsim>"
  Switch/1 -> [Pref]
  Product/1 -> DCL_LSC_LCL_Trafo_NoSwitching/2
  [Vref] -> Sum/2
  Sum/1 -> NotEqual3/1, NotEqual2/1, Saturation3/1
  Saturation3/1 -> NotEqual3/2, NotEqual2/2, [Vreflim]
  [Qavg_pu] -> Sum1/2
  [WTconsensus] -> Enabled/1
  Unit Delay10/1 -> [Vref]
  [QregBlockUp] -> PI_Std_AntiWindup_HoldUpDown_Backward/3
  Constant18/1 -> PI_Std_AntiWindup_HoldUpDown_Backward/4, PI_Std_AntiWindup_HoldUpDown_Backward/2, PI_Std_AntiWindup_HoldUpDown_Backward/6, PI_Std_AntiWindup_HoldUpDown_Backward/7
  [QregBlockDown] -> PI_Std_AntiWindup_HoldUpDown_Backward/5
  PI_Std_AntiWindup_HoldUpDown_Backward/7 -> Terminator1/1
  PI_Std_AntiWindup_HoldUpDown_Backward/6 -> Terminator6/1
  PI_Std_AntiWindup_HoldUpDown_Backward/5 -> Terminator7/1
  PI_Std_AntiWindup_HoldUpDown_Backward/4 -> Terminator8/1
  PI_Std_AntiWindup_HoldUpDown_Backward/3 -> Terminator9/1
  PI_Std_AntiWindup_HoldUpDown_Backward/2 -> Terminator10/1
  NotEqual2/1 -> Unit Delay12/1
  Unit Delay12/1 -> [QregBlockUp]
  NotEqual3/1 -> Unit Delay13/1
  Unit Delay13/1 -> [QregBlockDown]
  PI_Std_AntiWindup_HoldUpDown_Backward/1 -> Sum/1
  Bus Selector1/5 -> [WTconsensus]  "<WF_ReactiveConsensus>"
  Sum1/1 -> PI_Std_AntiWindup_HoldUpDown_Backward/1
  Enabled/1 -> Product1/2
  Enabled/2 -> Terminator12/1
  QavgWF/1 -> Product1/1
  Product1/1 -> Sum1/1
  connections:
  Controlled Current Source1/RConn1 -- DCL_LSC_LCL_Trafo_NoSwitching/LConn1
  DCL_LSC_LCL_Trafo_NoSwitching/RConn3 -- C/RConn1
  DCL_LSC_LCL_Trafo_NoSwitching/RConn1 -- A/RConn1
  DCL_LSC_LCL_Trafo_NoSwitching/RConn2 -- B/RConn1
  Controlled Current Source1/LConn1 -- DCL_LSC_LCL_Trafo_NoSwitching/LConn2

== system Just_The_Electrical_model/Electric system/Wind Farm/Wind Model Kaimal spectrum according to IEC61400-1 ==
  avg_wind : Inport
  Fcn : Fcn  Expr=turb_int*sqrt(L*u(1))/100/sqrt(2)
  Kaimal Filter : Subsystem
  Product : Product  SaturateOnIntegerOverflow=on  OutDataTypeStr=Inherit: Same as first input
  Scope : Scope  Commented=on  NumInputPorts=3
  Sum2 : Sum  SaturateOnIntegerOverflow=on  InputSameDT=on  OutDataTypeStr=Inherit: Same as first input
  White Noise_1 : Subsystem  mask(Continuous White Noise.){Cov=[1], Ts=T_sample, seed=WhiteNoiseSeed}
      mask prompts: Cov "Noise Power:"; Ts "Sample Time:"
      mask help:
      | White noise for continuous (s-domain) systems.
      | Band-limited using zero-order-hold.
      mask init:
      | r = rand(1,12); r2 = [r(1),r;r,r(12)]; t =[1:13;1:13];
      mask Help: Implemented using white noise into Zero-Order Hold block. The seed and power can be vectors of the same length to produce a vector of white noise sources. For faster simulation, set sample time to the highest value possible but in accordance with the fastest dynamics of system.
      mask Display: plot(t(:),r2(:))
  wind : Outport  InitialOutput=[u0]
  wires:
  Product/1 -> Sum2/1
  Sum2/1 -> wind/1  "wind"
  White Noise_1/1(Out_1) -> Scope/1, Kaimal Filter/2(In)
  Fcn/1 -> Scope/2, Product/1
  Kaimal Filter/1(Out) -> Scope/3, Product/2
  avg_wind/1 -> Sum2/2, Fcn/1, Kaimal Filter/1(avg_wind)

== system Just_The_Electrical_model/Electric system/Wind Farm/Wind Model Kaimal spectrum according to IEC61400-2 ==
  avg_wind : Inport
  Fcn : Fcn  Expr=turb_int*sqrt(L*u(1))/100/sqrt(2)
  Kaimal Filter : Subsystem
  Product : Product  SaturateOnIntegerOverflow=on  OutDataTypeStr=Inherit: Same as first input
  Sum2 : Sum  SaturateOnIntegerOverflow=on  InputSameDT=on  OutDataTypeStr=Inherit: Same as first input
  White Noise_1 : Subsystem  mask(Continuous White Noise.){Cov=[1], Ts=T_sample, seed=WhiteNoiseSeed}
      mask prompts: Cov "Noise Power:"; Ts "Sample Time:"
      mask help:
      | White noise for continuous (s-domain) systems.
      | Band-limited using zero-order-hold.
      mask init:
      | r = rand(1,12); r2 = [r(1),r;r,r(12)]; t =[1:13;1:13];
      mask Help: Implemented using white noise into Zero-Order Hold block. The seed and power can be vectors of the same length to produce a vector of white noise sources. For faster simulation, set sample time to the highest value possible but in accordance with the fastest dynamics of system.
      mask Display: plot(t(:),r2(:))
  wind : Outport  InitialOutput=[u0]
  wires:
  Product/1 -> Sum2/1
  Sum2/1 -> wind/1  "wind"
  White Noise_1/1(Out_1) -> Kaimal Filter/2(In)
  Fcn/1 -> Product/1
  Kaimal Filter/1(Out) -> Product/2
  avg_wind/1 -> Sum2/2, Fcn/1, Kaimal Filter/1(avg_wind)

== system Just_The_Electrical_model/Electric system/Wind Farm/Wind Model Kaimal spectrum according to IEC61400-3 ==
  avg_wind : Inport
  Fcn : Fcn  Expr=turb_int*sqrt(L*u(1))/100/sqrt(2)
  Kaimal Filter : Subsystem
  Product : Product  SaturateOnIntegerOverflow=on  OutDataTypeStr=Inherit: Same as first input
  Sum2 : Sum  SaturateOnIntegerOverflow=on  InputSameDT=on  OutDataTypeStr=Inherit: Same as first input
  White Noise_1 : Subsystem  mask(Continuous White Noise.){Cov=[1], Ts=T_sample, seed=WhiteNoiseSeed}
      mask prompts: Cov "Noise Power:"; Ts "Sample Time:"
      mask help:
      | White noise for continuous (s-domain) systems.
      | Band-limited using zero-order-hold.
      mask init:
      | r = rand(1,12); r2 = [r(1),r;r,r(12)]; t =[1:13;1:13];
      mask Help: Implemented using white noise into Zero-Order Hold block. The seed and power can be vectors of the same length to produce a vector of white noise sources. For faster simulation, set sample time to the highest value possible but in accordance with the fastest dynamics of system.
      mask Display: plot(t(:),r2(:))
  wind : Outport  InitialOutput=[u0]
  wires:
  Product/1 -> Sum2/1
  Sum2/1 -> wind/1  "wind"
  White Noise_1/1(Out_1) -> Kaimal Filter/2(In)
  Fcn/1 -> Product/1
  Kaimal Filter/1(Out) -> Product/2
  avg_wind/1 -> Sum2/2, Fcn/1, Kaimal Filter/1(avg_wind)

== system Just_The_Electrical_model/Electric system/rms and power calc/LP filter 1 ==
  in : Inport
  Discrete Transfer Fcn (with initial outputs) : simulink_extras/Additional Discrete/Discrete Transfer Fcn (with initial outputs)  N=[1/tau*Ts/2 1/tau*Ts/2]  D=[(1/tau*Ts/2+1) (1/tau*Ts/2-1)]  U0=x0  Y0=y0  TS=Ts
  out : Outport
  wires:
  Discrete Transfer Fcn (with initial outputs)/1 -> out/1
  in/1 -> Discrete Transfer Fcn (with initial outputs)/1

== system Just_The_Electrical_model/Electric system/rms and power calc/LP filter 66 ==
  in : Inport
  Discrete Transfer Fcn (with initial outputs) : simulink_extras/Additional Discrete/Discrete Transfer Fcn (with initial outputs)  N=[1/tau*Ts/2 1/tau*Ts/2]  D=[(1/tau*Ts/2+1) (1/tau*Ts/2-1)]  U0=x0  Y0=y0  TS=Ts
  out : Outport
  wires:
  Discrete Transfer Fcn (with initial outputs)/1 -> out/1
  in/1 -> Discrete Transfer Fcn (with initial outputs)/1

== system Just_The_Electrical_model/Electric system/rms and power calc/Low pass filter P1 ==
  in : Inport
  Discrete Transfer Fcn (with initial outputs) : simulink_extras/Additional Discrete/Discrete Transfer Fcn (with initial outputs)  N=[1/tau*Ts/2 1/tau*Ts/2]  D=[(1/tau*Ts/2+1) (1/tau*Ts/2-1)]  U0=x0  Y0=y0  TS=Ts
  out : Outport
  wires:
  Discrete Transfer Fcn (with initial outputs)/1 -> out/1
  in/1 -> Discrete Transfer Fcn (with initial outputs)/1

== system Just_The_Electrical_model/Electric system/rms and power calc/Low pass filter P2 ==
  in : Inport
  Discrete Transfer Fcn (with initial outputs) : simulink_extras/Additional Discrete/Discrete Transfer Fcn (with initial outputs)  N=[1/tau*Ts/2 1/tau*Ts/2]  D=[(1/tau*Ts/2+1) (1/tau*Ts/2-1)]  U0=x0  Y0=y0  TS=Ts
  out : Outport
  wires:
  Discrete Transfer Fcn (with initial outputs)/1 -> out/1
  in/1 -> Discrete Transfer Fcn (with initial outputs)/1

== system Just_The_Electrical_model/Electric system/rms and power calc/Low pass filter P3 ==
  in : Inport
  Discrete Transfer Fcn (with initial outputs) : simulink_extras/Additional Discrete/Discrete Transfer Fcn (with initial outputs)  N=[1/tau*Ts/2 1/tau*Ts/2]  D=[(1/tau*Ts/2+1) (1/tau*Ts/2-1)]  U0=x0  Y0=y0  TS=Ts
  out : Outport
  wires:
  in/1 -> Discrete Transfer Fcn (with initial outputs)/1
  Discrete Transfer Fcn (with initial outputs)/1 -> out/1

== system Just_The_Electrical_model/Electric system/rms and power calc/Low pass filter P4 ==
  in : Inport
  Discrete Transfer Fcn (with initial outputs) : simulink_extras/Additional Discrete/Discrete Transfer Fcn (with initial outputs)  N=[1/tau*Ts/2 1/tau*Ts/2]  D=[(1/tau*Ts/2+1) (1/tau*Ts/2-1)]  U0=x0  Y0=y0  TS=Ts
  out : Outport
  wires:
  in/1 -> Discrete Transfer Fcn (with initial outputs)/1
  Discrete Transfer Fcn (with initial outputs)/1 -> out/1

== system Just_The_Electrical_model/Electric system/rms and power calc/Low pass filter Q ==
  in : Inport
  Discrete Transfer Fcn (with initial outputs) : simulink_extras/Additional Discrete/Discrete Transfer Fcn (with initial outputs)  N=[1/tau*Ts/2 1/tau*Ts/2]  D=[(1/tau*Ts/2+1) (1/tau*Ts/2-1)]  U0=x0  Y0=y0  TS=Ts
  out : Outport
  wires:
  Discrete Transfer Fcn (with initial outputs)/1 -> out/1
  in/1 -> Discrete Transfer Fcn (with initial outputs)/1

== system Just_The_Electrical_model/Electric system/rms and power calc/Low pass filter Q1 ==
  in : Inport
  Discrete Transfer Fcn (with initial outputs) : simulink_extras/Additional Discrete/Discrete Transfer Fcn (with initial outputs)  N=[1/tau*Ts/2 1/tau*Ts/2]  D=[(1/tau*Ts/2+1) (1/tau*Ts/2-1)]  U0=x0  Y0=y0  TS=Ts
  out : Outport
  wires:
  Discrete Transfer Fcn (with initial outputs)/1 -> out/1
  in/1 -> Discrete Transfer Fcn (with initial outputs)/1

== system Just_The_Electrical_model/Electric system/rms and power calc/Low pass filter Q2 ==
  in : Inport
  Discrete Transfer Fcn (with initial outputs) : simulink_extras/Additional Discrete/Discrete Transfer Fcn (with initial outputs)  N=[1/tau*Ts/2 1/tau*Ts/2]  D=[(1/tau*Ts/2+1) (1/tau*Ts/2-1)]  U0=x0  Y0=y0  TS=Ts
  out : Outport
  wires:
  in/1 -> Discrete Transfer Fcn (with initial outputs)/1
  Discrete Transfer Fcn (with initial outputs)/1 -> out/1

== system Just_The_Electrical_model/Electric system/rms and power calc/Low pass filter Q3 ==
  in : Inport
  Discrete Transfer Fcn (with initial outputs) : simulink_extras/Additional Discrete/Discrete Transfer Fcn (with initial outputs)  N=[1/tau*Ts/2 1/tau*Ts/2]  D=[(1/tau*Ts/2+1) (1/tau*Ts/2-1)]  U0=x0  Y0=y0  TS=Ts
  out : Outport
  wires:
  in/1 -> Discrete Transfer Fcn (with initial outputs)/1
  Discrete Transfer Fcn (with initial outputs)/1 -> out/1

== system Just_The_Electrical_model/Electric system/Automatic voltage regulator/PID_Governor1/LP filter power ==
  in : Inport
  Discrete Transfer Fcn (with initial outputs) : simulink_extras/Additional Discrete/Discrete Transfer Fcn (with initial outputs)  N=[1/tau*Ts/2 1/tau*Ts/2]  D=[(1/tau*Ts/2+1) (1/tau*Ts/2-1)]  U0=x0  Y0=y0  TS=Ts
  out : Outport
  wires:
  Discrete Transfer Fcn (with initial outputs)/1 -> out/1
  in/1 -> Discrete Transfer Fcn (with initial outputs)/1

== system Just_The_Electrical_model/Electric system/SM_simple/powerCalcAndFilt1/LP filter frequency1 ==
  in : Inport
  Discrete Transfer Fcn (with initial outputs) : simulink_extras/Additional Discrete/Discrete Transfer Fcn (with initial outputs)  N=[1/tau*Ts/2 1/tau*Ts/2]  D=[(1/tau*Ts/2+1) (1/tau*Ts/2-1)]  U0=x0  Y0=y0  TS=Ts
  out : Outport
  wires:
  Discrete Transfer Fcn (with initial outputs)/1 -> out/1
  in/1 -> Discrete Transfer Fcn (with initial outputs)/1

== system Just_The_Electrical_model/Electric system/SM_simple/powerCalcAndFilt1/LP filter frequency2 ==
  in : Inport
  Discrete Transfer Fcn (with initial outputs) : simulink_extras/Additional Discrete/Discrete Transfer Fcn (with initial outputs)  N=[1/tau*Ts/2 1/tau*Ts/2]  D=[(1/tau*Ts/2+1) (1/tau*Ts/2-1)]  U0=x0  Y0=y0  TS=Ts
  out : Outport
  wires:
  Discrete Transfer Fcn (with initial outputs)/1 -> out/1
  in/1 -> Discrete Transfer Fcn (with initial outputs)/1

== system Just_The_Electrical_model/Electric system/Wind Farm/Wind Model Kaimal spectrum according to IEC61400-1/Kaimal Filter ==
  avg_wind : Inport
  In : Inport  Port=2
  A/D : Gain  Gain=0.0182/1.3463  SaturateOnIntegerOverflow=on  OutDataTypeStr=Inherit: Same as input  ParamDataTypeStr=Inherit: Same as input
  Coefficients : Subsystem
  Integrator : Integrator
  Integrator1 : Integrator
  Product{,1..3} (4 alike) : Product  SaturateOnIntegerOverflow=on  OutDataTypeStr=Inherit: Same as first input
  Sum : Sum  Inputs=|++  SaturateOnIntegerOverflow=on
  Sum1 : Sum  Inputs=++-  SaturateOnIntegerOverflow=on
  Sum2 : Sum  Inputs=+|-  SaturateOnIntegerOverflow=on
  Out : Outport
  wires:
  avg_wind/1 -> Coefficients/1(avg_wind)
  Coefficients/4(FD) -> [FD]
  Coefficients/3(ED) -> [ED]
  Coefficients/2(CD) -> [CD]
  Coefficients/1(BD) -> [BD]
  [FD] -> Product3/2
  [ED] -> Product2/2
  [CD] -> Product1/2
  [BD] -> Product/2
  In/1 -> Product1/1, Product/1, A/D/1
  Sum/1 -> Out/1, Product3/1, Product2/1
  Product1/1 -> Sum2/1
  Product3/1 -> Sum2/2
  Sum2/1 -> Integrator1/1
  Product2/1 -> Sum1/3
  Integrator1/1 -> Sum1/2
  Product/1 -> Sum1/1
  Sum1/1 -> Integrator/1
  Integrator/1 -> Sum/2
  A/D/1 -> Sum/1

== system Just_The_Electrical_model/Electric system/Wind Farm/Wind Model Kaimal spectrum according to IEC61400-1/White Noise_1 ==
  Gain : Gain  Gain=[sqrt(Cov)]/[sqrt(Ts)]  SaturateOnIntegerOverflow=on  OutDataTypeStr=Inherit: Same as input  ParamDataTypeStr=Inherit: Same as input
  White Noise : RandomNumber  Seed=seed  SampleTime=Ts
  Zero-Order Hold : ZeroOrderHold  SampleTime=Ts
  Out_1 : Outport
  wires:
  White Noise/1 -> Zero-Order Hold/1
  Gain/1 -> Out_1/1
  Zero-Order Hold/1 -> Gain/1

== system Just_The_Electrical_model/Electric system/Wind Farm/Wind Model Kaimal spectrum according to IEC61400-2/Kaimal Filter ==
  avg_wind : Inport
  In : Inport  Port=2
  A/D : Gain  Gain=0.0182/1.3463  SaturateOnIntegerOverflow=on  OutDataTypeStr=Inherit: Same as input  ParamDataTypeStr=Inherit: Same as input
  Coefficients : Subsystem
  Integrator : Integrator
  Integrator1 : Integrator
  Product{,1..3} (4 alike) : Product  SaturateOnIntegerOverflow=on  OutDataTypeStr=Inherit: Same as first input
  Sum : Sum  Inputs=|++  SaturateOnIntegerOverflow=on
  Sum1 : Sum  Inputs=++-  SaturateOnIntegerOverflow=on
  Sum2 : Sum  Inputs=+|-  SaturateOnIntegerOverflow=on
  Out : Outport
  wires:
  avg_wind/1 -> Coefficients/1(avg_wind)
  Coefficients/4(FD) -> [FD]
  Coefficients/3(ED) -> [ED]
  Coefficients/2(CD) -> [CD]
  Coefficients/1(BD) -> [BD]
  [FD] -> Product3/2
  [ED] -> Product2/2
  [CD] -> Product1/2
  [BD] -> Product/2
  In/1 -> Product1/1, Product/1, A/D/1
  Sum/1 -> Out/1, Product3/1, Product2/1
  Product1/1 -> Sum2/1
  Product3/1 -> Sum2/2
  Sum2/1 -> Integrator1/1
  Product2/1 -> Sum1/3
  Integrator1/1 -> Sum1/2
  Product/1 -> Sum1/1
  Sum1/1 -> Integrator/1
  Integrator/1 -> Sum/2
  A/D/1 -> Sum/1

== system Just_The_Electrical_model/Electric system/Wind Farm/Wind Model Kaimal spectrum according to IEC61400-2/White Noise_1 ==
  Gain : Gain  Gain=[sqrt(Cov)]/[sqrt(Ts)]  SaturateOnIntegerOverflow=on  OutDataTypeStr=Inherit: Same as input  ParamDataTypeStr=Inherit: Same as input
  White Noise : RandomNumber  Seed=seed  SampleTime=Ts
  Zero-Order Hold : ZeroOrderHold  SampleTime=Ts
  Out_1 : Outport
  wires:
  White Noise/1 -> Zero-Order Hold/1
  Gain/1 -> Out_1/1
  Zero-Order Hold/1 -> Gain/1

== system Just_The_Electrical_model/Electric system/Wind Farm/Wind Model Kaimal spectrum according to IEC61400-3/Kaimal Filter ==
  avg_wind : Inport
  In : Inport  Port=2
  A/D : Gain  Gain=0.0182/1.3463  SaturateOnIntegerOverflow=on  OutDataTypeStr=Inherit: Same as input  ParamDataTypeStr=Inherit: Same as input
  Coefficients : Subsystem
  Integrator : Integrator
  Integrator1 : Integrator
  Product{,1..3} (4 alike) : Product  SaturateOnIntegerOverflow=on  OutDataTypeStr=Inherit: Same as first input
  Sum : Sum  Inputs=|++  SaturateOnIntegerOverflow=on
  Sum1 : Sum  Inputs=++-  SaturateOnIntegerOverflow=on
  Sum2 : Sum  Inputs=+|-  SaturateOnIntegerOverflow=on
  Out : Outport
  wires:
  avg_wind/1 -> Coefficients/1(avg_wind)
  Coefficients/4(FD) -> [FD]
  Coefficients/3(ED) -> [ED]
  Coefficients/2(CD) -> [CD]
  Coefficients/1(BD) -> [BD]
  [FD] -> Product3/2
  [ED] -> Product2/2
  [CD] -> Product1/2
  [BD] -> Product/2
  In/1 -> Product1/1, Product/1, A/D/1
  Sum/1 -> Out/1, Product3/1, Product2/1
  Product1/1 -> Sum2/1
  Product3/1 -> Sum2/2
  Sum2/1 -> Integrator1/1
  Product2/1 -> Sum1/3
  Integrator1/1 -> Sum1/2
  Product/1 -> Sum1/1
  Sum1/1 -> Integrator/1
  Integrator/1 -> Sum/2
  A/D/1 -> Sum/1

== system Just_The_Electrical_model/Electric system/Wind Farm/Wind Model Kaimal spectrum according to IEC61400-3/White Noise_1 ==
  Gain : Gain  Gain=[sqrt(Cov)]/[sqrt(Ts)]  SaturateOnIntegerOverflow=on  OutDataTypeStr=Inherit: Same as input  ParamDataTypeStr=Inherit: Same as input
  White Noise : RandomNumber  Seed=seed  SampleTime=Ts
  Zero-Order Hold : ZeroOrderHold  SampleTime=Ts
  Out_1 : Outport
  wires:
  White Noise/1 -> Zero-Order Hold/1
  Gain/1 -> Out_1/1
  Zero-Order Hold/1 -> Gain/1

== system Just_The_Electrical_model/Electric system/Wind Farm/Wind Model Kaimal spectrum according to IEC61400-1/Kaimal Filter/Coefficients ==
  avg_wind : Inport
  BD coeff : Fcn  Expr=1.3653/1.3463/(L/2/pi/u(1))
  CD coeff : Fcn  Expr=0.9846/1.3463/(L/2/pi/u(1))^2
  ED coeff : Fcn  Expr=3.7593/1.3463/(L/2/pi/u(1))
  FD coeff : Fcn  Expr=1/1.3463/(L/2/pi/u(1))^2
  BD : Outport
  CD : Outport  Port=2
  ED : Outport  Port=3
  FD : Outport  Port=4
  wires:
  FD coeff/1 -> FD/1
  ED coeff/1 -> ED/1
  CD coeff/1 -> CD/1
  BD coeff/1 -> BD/1
  avg_wind/1 -> FD coeff/1, ED coeff/1, CD coeff/1, BD coeff/1

== system Just_The_Electrical_model/Electric system/Wind Farm/Wind Model Kaimal spectrum according to IEC61400-2/Kaimal Filter/Coefficients ==
  avg_wind : Inport
  BD coeff : Fcn  Expr=1.3653/1.3463/(L/2/pi/u(1))
  CD coeff : Fcn  Expr=0.9846/1.3463/(L/2/pi/u(1))^2
  ED coeff : Fcn  Expr=3.7593/1.3463/(L/2/pi/u(1))
  FD coeff : Fcn  Expr=1/1.3463/(L/2/pi/u(1))^2
  BD : Outport
  CD : Outport  Port=2
  ED : Outport  Port=3
  FD : Outport  Port=4
  wires:
  FD coeff/1 -> FD/1
  ED coeff/1 -> ED/1
  CD coeff/1 -> CD/1
  BD coeff/1 -> BD/1
  avg_wind/1 -> FD coeff/1, ED coeff/1, CD coeff/1, BD coeff/1

== system Just_The_Electrical_model/Electric system/Wind Farm/Wind Model Kaimal spectrum according to IEC61400-3/Kaimal Filter/Coefficients ==
  avg_wind : Inport
  BD coeff : Fcn  Expr=1.3653/1.3463/(L/2/pi/u(1))
  CD coeff : Fcn  Expr=0.9846/1.3463/(L/2/pi/u(1))^2
  ED coeff : Fcn  Expr=3.7593/1.3463/(L/2/pi/u(1))
  FD coeff : Fcn  Expr=1/1.3463/(L/2/pi/u(1))^2
  BD : Outport
  CD : Outport  Port=2
  ED : Outport  Port=3
  FD : Outport  Port=4
  wires:
  FD coeff/1 -> FD/1
  ED coeff/1 -> ED/1
  CD coeff/1 -> CD/1
  BD coeff/1 -> BD/1
  avg_wind/1 -> FD coeff/1, ED coeff/1, CD coeff/1, BD coeff/1
